simulink model "test_envelope"  (R2024b)
settings: Solver=FixedStepAuto  StartTime=0.0  StopTime=5  FixedStep=0.01  RelTol=1e-3
settings Model: Creator=Thoma  LastModifiedBy=Thoma

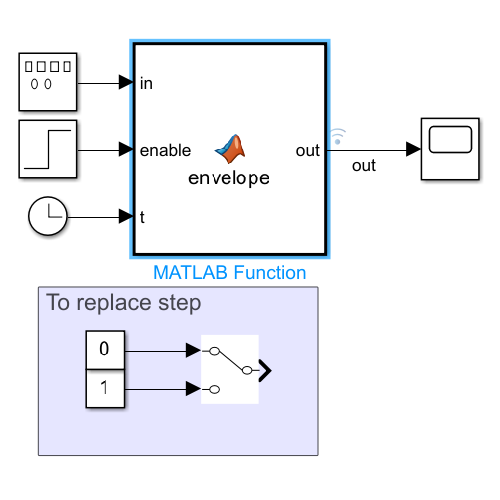
[thumbnail: Simulink's stored preview of the top-level diagram]
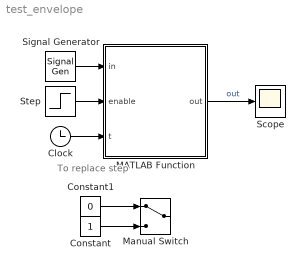
== system test_envelope ==
  note: To replace step
  Clock : Clock
  Constant : Constant
  Constant1 : Constant  Value=0
  MATLAB Function : MATLAB Function  TreatAsAtomicUnit=on
  Manual Switch : ManualSwitch
  Scope : Scope
  Signal Generator : SignalGenerator
  Step : Step  Time=1.2  SampleTime=0
  wires:
  Constant/1 -> Manual Switch/2
  Constant1/1 -> Manual Switch/1
  Step/1 -> MATLAB Function/2(enable)
  Signal Generator/1 -> MATLAB Function/1(in)
  MATLAB Function/1(out) -> Scope/1  "out"
  Clock/1 -> MATLAB Function/3(t)

== matlab function test_envelope/MATLAB Function ==
  data: in input; out output; enable input; t input
function out = envelope(in, enable,t)
    % Envelope for testing
    T = 2; % [sec]
    persistent t0
    
    if isempty(t0)
        t0 = 0;
    end

    if enable
        if t0 == 0
            t0 = t;
        end
        tau = min(max((t-t0) / T, 0), 1);
        out = in*(3*tau^2 - 2*tau^3);
    else
        out = 0;
        t0 = 0;
    end
end
